simulink model "BF_sans_controleur_analyse"  (R2021b)
settings: Solver=VariableStepAuto  StartTime=0.0  StopTime=10.0  RelTol=1e-3
values from neighbouring files (symbols this model uses):
  A = [0 0 0  1 0 0   0 0 0   0 0 0 ... (first row only)    [main.m]
  B = [0 0 0 0 ... (first row only)    [main.m]
  B2 = [0 0 ... (first row only)    [main.m]
  C = eye(12)    [main.m]
  C_control = [C(1:7,:);C(9:12,:)]    [main.m]
  D = zeros(12,6)    [main.m]
  F = [1,0;1,0;0,1;0,1]    [main.m]
  H_val = H_val.D    [main.m]
  K_val = K_val.D    [main.m]
undefined symbols (not defined in the file or in its folder): x_6
settings Model: Creator=florian  LastModifiedBy=florian

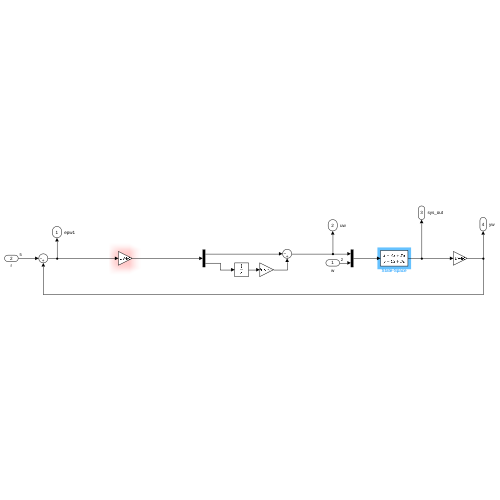
[thumbnail: Simulink's stored preview of the top-level diagram]
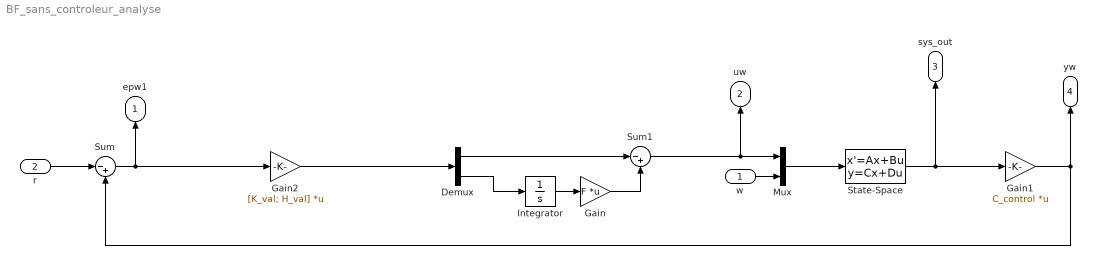
== system BF_sans_controleur_analyse ==
  w : Inport  PortDimensions=2
  r : Inport  Port=2  PortDimensions=5
  Demux : Demux  Outputs=2
  Gain : Gain  Gain=F  Multiplication=Matrix(K*u) (u vector)
  Gain1 : Gain  Gain=C_control  Multiplication=Matrix(K*u) (u vector)
  Gain2 : Gain  Gain=[K_val; H_val]  Multiplication=Matrix(K*u) (u vector)
  Integrator : Integrator
  Mux : Mux  Inputs=2
  State-Space : StateSpace  A=A  B=[B, B2]  C=C  D=D  InitialCondition=x_6
  Sum : Sum  Inputs=|-+
  Sum1 : Sum  Inputs=|-+
  epw1 : Outport  InitialOutput=0
  uw : Outport  Port=2  InitialOutput=0
  sys_out : Outport  Port=3
  yw : Outport  Port=4
  wires:
  Demux/2 -> Integrator/1
  Sum1/1 -> uw/1, Mux/1
  Sum/1 -> Gain2/1, epw1/1
  Gain2/1 -> Demux/1
  State-Space/1 -> Gain1/1, sys_out/1
  Gain/1 -> Sum1/2
  w/1 -> Mux/2
  Gain1/1 -> yw/1, Sum/2
  Demux/1 -> Sum1/1
  Mux/1 -> State-Space/1
  r/1 -> Sum/1
  Integrator/1 -> Gain/1
